simulink model "model"  (R2018a)
settings: Solver=VariableStepAuto  StartTime=0.0  StopTime=20  MaxStep=0.01  RelTol=1e-8  EnableMultiTasking=on
settings Model: Creator=Pracownik  LastModifiedBy=CHADI
settings DataIOCC: LimitDataPoints=on
settings OptimizationCC: LifeSpan=inf
settings DebuggingCC: AllowSymbolicDim=off  SFUnexpectedBacktrackingDiag=warning  SFNoUnconditionalDefaultTransitionDiag=warning  SFExecutionAtInitializationDiag=none
settings ModelReferenceCC: PropagateSignalLabelsOutOfModel=off
settings CodeAppCC: StateflowObjectComments=on
settings GRTTargetCC: TargetLangStandard=C89/C90 (ANSI)
settings ConfigComp: CovMetricSettings=dw  CovHtmlReporting=on  CovSaveCumulativeToWorkspaceVar=on  CovSaveSingleToWorkspaceVar=on  CovExternalEMLEnable=off

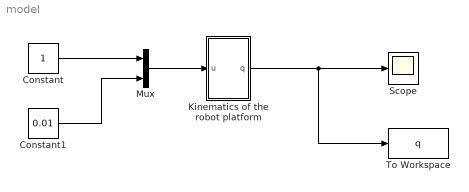
== system model ==
  Constant : Constant
  Constant1 : Constant  Value=0.01
  Kinematics of the robot platform : Subsystem
  Mux : Mux  Inputs=2
  Scope : Scope
  To Workspace : ToWorkspace  VariableName=q  SampleTime=-1
  wires:
  Kinematics of the robot platform/1(q) -> To Workspace/1, Scope/1
  Mux/1 -> Kinematics of the robot platform/1(u)
  Constant/1 -> Mux/1
  Constant1/1 -> Mux/2

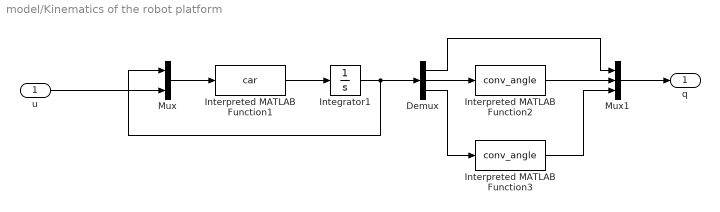
== system model/Kinematics of the robot platform ==
  u : Inport
  Demux : Demux  Outputs=[2 1 1]
  Integrator1 : Integrator  InitialCondition=[0; 0; 0; 0]
  Interpreted MATLAB Function1 : MATLABFcn  MATLABFcn=car
  Interpreted MATLAB Function2 : MATLABFcn  MATLABFcn=conv_angle
  Interpreted MATLAB Function3 : MATLABFcn  MATLABFcn=conv_angle
  Mux : Mux  Inputs=[4 2]
  Mux1 : Mux  Inputs=[2 1 1]
  q : Outport
  wires:
  Mux/1 -> Interpreted MATLAB Function1/1
  Interpreted MATLAB Function1/1 -> Integrator1/1
  Integrator1/1 -> Demux/1, Mux/1
  u/1 -> Mux/2
  Demux/2 -> Interpreted MATLAB Function2/1
  Interpreted MATLAB Function2/1 -> Mux1/2
  Demux/1 -> Mux1/1
  Mux1/1 -> q/1
  Demux/3 -> Interpreted MATLAB Function3/1
  Interpreted MATLAB Function3/1 -> Mux1/3
